simulink model "Parent_Mobile"  (R2023a)
settings: Solver=FixedStepDiscrete  StartTime=0.0  StopTime=inf  RelTol=1e-3
undefined symbols (not defined in the file): Alt, Child_Safety, Lat, Lon, ThingSpeak_X_Acc, X_Acc, X_Gyro, Y_Acc, Y_Gyro, Z_Acc, Z_Gyro
libraries: androidcommunicationlib x16, androiduilib x13, androidsensorlib x7, androidaudiovideolib x5
settings Model: Creator=dhart  LastModifiedBy=dhart
settings OptimizationCC: EnhancedBackFolding=on  PassReuseOutputArgsAs=Individual arguments  ZeroExternalMemoryAtStartup=off  ZeroInternalMemoryAtStartup=off  MaxStackSize=64  OptimizeBlockOrder=speed  DifferentSizesBufferReuse=on  OptimizationCustomize=off  EfficientTunableParamExpr=on
settings DebuggingCC: ParameterTunabilityLossMsg=error
settings HardwareCC: ProdBitPerPointer=32  ProdBitPerSizeT=32  ProdBitPerPtrDiffT=32  ProdLargestAtomicInteger=Long  ProdLargestAtomicFloat=Double  ProdWordSize=32  ProdHWDeviceType=ARM Compatible->ARM Cortex
settings SFSimCC: MATLABDynamicMemAlloc=off
settings RTWCC: Description=Embedded Coder  SystemTargetFile=ert.tlc  HardwareBoard=Android Device  TLCOptions="-aInlineSetEventsForThisBaseRateFcn=TLC_FALSE -aSuppressMultiTaskScheduler=TLC_FALSE  -aRateBasedStepFcn=0"  TemplateMakefile=ert_default_tmf  RTWVerbose=off  Toolchain=Android SDK/NDK Tools  BuildConfiguration=Faster Runs
settings CodeAppCC: ForceParamTrailComments=on  IgnoreCustomStorageClasses=off  OperatorAnnotations=on  SimulinkDataObjDesc=on  SFDataObjDesc=on  InsertBlockDesc=on

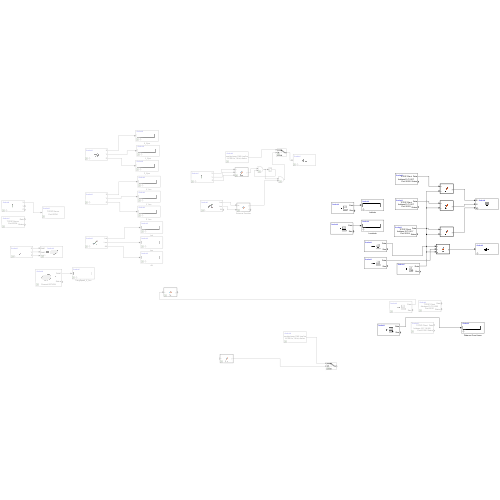
[thumbnail: Simulink's stored preview of the top-level diagram]
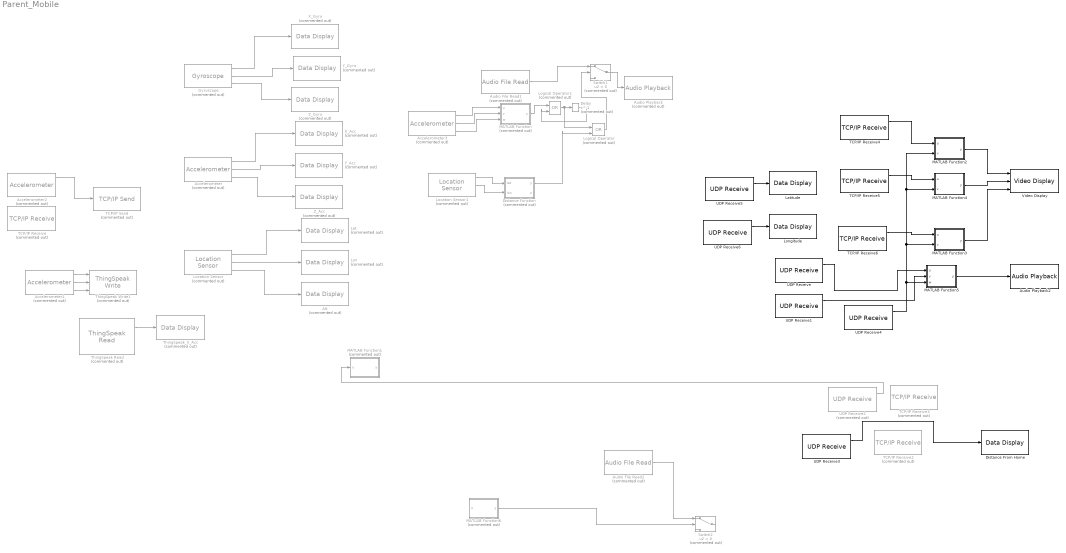
== system Parent_Mobile ==
  Accelerometer{,1..3} (4 alike) : androidsensorlib/Accelerometer  Commented=on  OutputVector=off  SampleTime=0.1  BlockPlatform=Android
  Alt : androiduilib/Data Display  Commented=on  DataDisplayId=Child_Safety/Alt  Format=Float  Precision=6  SimulateUsing=Code generation  blockPlatform=Android
  Audio File Read1 : androidaudiovideolib/Audio File Read  Commented=on  FileName=C:\Users\dhart\Downloads\mixkit-censorship-beep-1082 (mp3cut.net).wav  FrameSize=4410
  Audio File Read2 : androidaudiovideolib/Audio File Read  Commented=on  FileName=C:\Users\dhart\Downloads\mixkit-censorship-beep-1082 (mp3cut.net).wav  FrameSize=4410
  Audio Playback : androidaudiovideolib/Audio Playback  Commented=on  SampleFreq=44100  AudioSamplingFreq=44100  SampleTime=0.1  DeviceStr=0  QueueDuration=0  BlockPlatform=Android
  Audio Playback2 : androidaudiovideolib/Audio Playback  SampleFreq=44100  AudioSamplingFreq=44100  SampleTime=0.1  DeviceStr=0  QueueDuration=0  BlockPlatform=Android
  Delay : Delay  Commented=on  DelayLength=1  InitialCondition=0
  Distance From Home : androiduilib/Data Display  DataDisplayId=Parent_Mobile/Distance_From_Home  Format=Float  Precision=6  SimulateUsing=Code generation  blockPlatform=Android
  Distance Function : MATLAB Function  Commented=on  TreatAsAtomicUnit=on
  Gyroscope : androidsensorlib/Gyroscope  Commented=on  OutputVector=off  SampleTime=0.1  BlockPlatform=Android
  Lat : androiduilib/Data Display  Commented=on  DataDisplayId=Child_Safety/Lat  Format=Float  Precision=6  SimulateUsing=Code generation  blockPlatform=Android
  Latitude : androiduilib/Data Display  DataDisplayId=Parent_Mobile/Latitude  Format=Float  Precision=6  SimulateUsing=Code generation  blockPlatform=Android
  Location Sensor : androidsensorlib/Location Sensor  Commented=on  OutputVector=off  SampleTime=0.1  BlockPlatform=Android
  Location Sensor1 : androidsensorlib/Location Sensor  Commented=on  OutputVector=off  SampleTime=0.1  BlockPlatform=Android
  Logical Operator : Logic  Commented=on  Operator=OR  IconShape=distinctive  AllPortsSameDT=off  OutDataTypeStr=boolean
  Logical Operator1 : Logic  Commented=on  Operator=OR  IconShape=distinctive  AllPortsSameDT=off  OutDataTypeStr=boolean
  Lon : androiduilib/Data Display  Commented=on  DataDisplayId=Child_Safety/Lon  Format=Float  Precision=6  SimulateUsing=Code generation  blockPlatform=Android
  Longitude : androiduilib/Data Display  DataDisplayId=Parent_Mobile/Longitude  Format=Float  Precision=6  SimulateUsing=Code generation  blockPlatform=Android
  MATLAB Function : MATLAB Function  Commented=on  TreatAsAtomicUnit=on
  MATLAB Function1 : MATLAB Function  Commented=on  TreatAsAtomicUnit=on
  MATLAB Function2 : MATLAB Function  TreatAsAtomicUnit=on
  MATLAB Function3 : MATLAB Function  TreatAsAtomicUnit=on
  MATLAB Function4 : MATLAB Function  TreatAsAtomicUnit=on
  MATLAB Function5 : MATLAB Function  TreatAsAtomicUnit=on
  MATLAB Function6 : MATLAB Function  Commented=on  TreatAsAtomicUnit=on
  Switch1 : Switch  Commented=on  Criteria=u2 > Threshold  SaturateOnIntegerOverflow=off  InputSameDT=off
  Switch2 : Switch  Commented=on  Criteria=u2 > Threshold  SaturateOnIntegerOverflow=off  InputSameDT=off
  TCP/IP Receive : androidcommunicationlib/TCP//IP Receive  Commented=on  TCPReceiveId=Child_Safety/TCP//IP_Receive  Mode_=Server  LocalServerPort_=25784  RemoteAddr_=127.0.0.1  RemoteServerPort_=25000  DataType_=uint8  DataSize_=1  SampleTime_=0.1  ClientPortBindingSelection_=off  ClientPortToBind_=35000  BlockingMode_=off  BlockTimeout_=0.1
  TCP/IP Receive2 : androidcommunicationlib/TCP//IP Receive  Commented=on  TCPReceiveId=Parent_Mobile/TCP//IP_Receive2  Mode_=Client  LocalServerPort_=25000  RemoteAddr_=10.7.18.205  RemoteServerPort_=25150  DataType_=int16  DataSize_=1  SampleTime_=0.1  ClientPortBindingSelection_=off  ClientPortToBind_=35000  BlockingMode_=off  BlockTimeout_=0.1
  TCP/IP Receive3 : androidcommunicationlib/TCP//IP Receive  Commented=on  TCPReceiveId=Parent_Mobile/TCP//IP_Receive3  Mode_=Client  LocalServerPort_=25000  RemoteAddr_=10.7.18.205  RemoteServerPort_=25151  DataType_=int16  DataSize_=4410  SampleTime_=0.1  ClientPortBindingSelection_=off  ClientPortToBind_=35000  BlockingMode_=off  BlockTimeout_=0.1
  TCP/IP Receive4 : androidcommunicationlib/TCP//IP Receive  TCPReceiveId=Parent_Mobile/TCP//IP_Receive4  Mode_=Client  LocalServerPort_=25000  RemoteAddr_=10.7.2.217  RemoteServerPort_=39152  DataType_=uint8  DataSize_=76800  SampleTime_=2  ClientPortBindingSelection_=off  ClientPortToBind_=35000  BlockingMode_=off  BlockTimeout_=0.1
  TCP/IP Receive5 : androidcommunicationlib/TCP//IP Receive  TCPReceiveId=Parent_Mobile/TCP//IP_Receive5  Mode_=Client  LocalServerPort_=25000  RemoteAddr_=10.7.2.217  RemoteServerPort_=39153  DataType_=uint8  DataSize_=76800  SampleTime_=2  ClientPortBindingSelection_=off  ClientPortToBind_=35000  BlockingMode_=off  BlockTimeout_=0.1
  TCP/IP Receive6 : androidcommunicationlib/TCP//IP Receive  TCPReceiveId=Parent_Mobile/TCP//IP_Receive6  Mode_=Client  LocalServerPort_=25000  RemoteAddr_=10.7.2.217  RemoteServerPort_=39154  DataType_=uint8  DataSize_=76800  SampleTime_=2  ClientPortBindingSelection_=off  ClientPortToBind_=35000  BlockingMode_=off  BlockTimeout_=0.1
  TCP/IP Send : androidcommunicationlib/TCP//IP Send  Commented=on  TCPSendId=Child_Safety/TCP//IP_Send  Mode_=Server  LocalServerPort_=25784  RemoteAddr_=127.0.0.1  RemoteServerPort_=25498  ClientPortBindingSelection_=off  ClientPortToBind_=35000  BlockingMode_=off  BlockTimeout_=0.1
  ThingSpeak Read : androidcommunicationlib/ThingSpeak Read  Commented=on  ChannelID=2273034  ChannelAccess=Private  ReadAPIKey=WXUH9J7EYEMDF8NM  FieldNumber=1  SampleTime=0.1
  ThingSpeak Write1 : androidcommunicationlib/ThingSpeak Write  Commented=on  ChannelID=2273034  WriteAPIKey=W5LD3WN1B2LJ7SVE  NumberOfFields=3  UpdateInterval=15  LocationEnabled=off  LocationSource=Block dialog  BlockPlatform=Android
  ThingSpeak_X_Acc : androiduilib/Data Display  Commented=on  DataDisplayId=Child_Safety/ThingSpeak_X_Acc  Format=Float  Precision=6  SimulateUsing=Code generation  blockPlatform=Android
  UDP Receive : androidcommunicationlib/UDP Receive  localURL='0.0.0.0'  localPort=39155  remoteURL='0.0.0.0'  remotePort=-1  recvBufferSize=8192  signalDatatype=int16  dims=4410  isVarSize=off  showBlockingTime=off  blockingTime=0  sampletime=0.1  blockPlatform=Android
  UDP Receive1 : androidcommunicationlib/UDP Receive  localURL='0.0.0.0'  localPort=39156  remoteURL='0.0.0.0'  remotePort=-1  recvBufferSize=8192  signalDatatype=int16  dims=4410  isVarSize=off  showBlockingTime=off  blockingTime=0  sampletime=0.1  blockPlatform=Android
  UDP Receive2 : androidcommunicationlib/UDP Receive  Commented=on  localURL='0.0.0.0'  localPort=25151  remoteURL='0.0.0.0'  remotePort=-1  recvBufferSize=8192  signalDatatype=int16  dims=4410  isVarSize=off  showBlockingTime=off  blockingTime=0  sampletime=0.1  blockPlatform=Android
  UDP Receive3 : androidcommunicationlib/UDP Receive  localURL='0.0.0.0'  localPort=39150  remoteURL='0.0.0.0'  remotePort=-1  recvBufferSize=8192  signalDatatype=double  dims=1  isVarSize=off  showBlockingTime=off  blockingTime=0  sampletime=0.1  blockPlatform=Android
  UDP Receive4 : androidcommunicationlib/UDP Receive  localURL='0.0.0.0'  localPort=39157  remoteURL='0.0.0.0'  remotePort=-1  recvBufferSize=8192  signalDatatype=single  dims=1  isVarSize=off  showBlockingTime=off  blockingTime=0  sampletime=0.1  blockPlatform=Android
  UDP Receive5 : androidcommunicationlib/UDP Receive  localURL='0.0.0.0'  localPort=39158  remoteURL='0.0.0.0'  remotePort=-1  recvBufferSize=8192  signalDatatype=double  dims=1  isVarSize=off  showBlockingTime=off  blockingTime=0  sampletime=0.1  blockPlatform=Android
  UDP Receive6 : androidcommunicationlib/UDP Receive  localURL='0.0.0.0'  localPort=39159  remoteURL='0.0.0.0'  remotePort=-1  recvBufferSize=8192  signalDatatype=double  dims=1  isVarSize=off  showBlockingTime=off  blockingTime=0  sampletime=0.1  blockPlatform=Android
  Video Display : androidaudiovideolib/Video Display  BlockPlatform=Android
  X_Acc : androiduilib/Data Display  Commented=on  DataDisplayId=Child_Safety/X_Acc  Format=Float  Precision=6  SimulateUsing=Code generation  blockPlatform=Android
  X_Gyro : androiduilib/Data Display  Commented=on  DataDisplayId=Child_Safety/X_Gyro  Format=Float  Precision=6  SimulateUsing=Code generation  blockPlatform=Android
  Y_Acc : androiduilib/Data Display  Commented=on  DataDisplayId=Child_Safety/Y_Acc  Format=Float  Precision=6  SimulateUsing=Code generation  blockPlatform=Android
  Y_Gyro : androiduilib/Data Display  Commented=on  DataDisplayId=Child_Safety/Y_Gyro  Format=Float  Precision=6  SimulateUsing=Code generation  blockPlatform=Android
  Z_Acc : androiduilib/Data Display  Commented=on  DataDisplayId=Child_Safety/Z_Acc  Format=Float  Precision=6  SimulateUsing=Code generation  blockPlatform=Android
  Z_Gyro : androiduilib/Data Display  Commented=on  DataDisplayId=Child_Safety/Z_Gyro  Format=Float  Precision=6  SimulateUsing=Code generation  blockPlatform=Android
  wires:
  Accelerometer/1 -> X_Acc/1
  Accelerometer/2 -> Y_Acc/1
  Accelerometer/3 -> Z_Acc/1
  Location Sensor/2 -> Lon/1
  Location Sensor/3 -> Alt/1
  Gyroscope/1 -> X_Gyro/1
  Gyroscope/2 -> Y_Gyro/1
  Gyroscope/3 -> Z_Gyro/1
  Location Sensor/1 -> Lat/1
  Location Sensor1/1 -> Distance Function/1(lat)
  Location Sensor1/2 -> Distance Function/2(lon)
  Accelerometer1/1 -> ThingSpeak Write1/1
  Accelerometer1/2 -> ThingSpeak Write1/2
  Accelerometer1/3 -> ThingSpeak Write1/3
  Accelerometer2/1 -> TCP/IP Send/1
  ThingSpeak Read/1 -> ThingSpeak_X_Acc/1
  Accelerometer3/1 -> MATLAB Function/1(u)
  Accelerometer3/2 -> MATLAB Function/2(v)
  Accelerometer3/3 -> MATLAB Function/3(w)
  Audio File Read1/1 -> Switch1/1
  Switch1/1 -> Audio Playback/1
  Distance Function/1(y) -> Logical Operator/2
  Logical Operator/1 -> Switch1/2
  MATLAB Function/1(y) -> Logical Operator1/1
  Logical Operator1/1 -> Logical Operator/1, Delay/1
  Delay/1 -> Logical Operator1/2
  MATLAB Function2/1(y) -> Video Display/1
  MATLAB Function4/1(y) -> Video Display/2
  MATLAB Function3/1(y) -> Video Display/3
  MATLAB Function5/1(y) -> Audio Playback2/1
  UDP Receive/1 -> MATLAB Function5/1(u)
  UDP Receive1/1 -> MATLAB Function5/2(v)
  TCP/IP Receive4/1 -> MATLAB Function2/1(u)
  TCP/IP Receive5/1 -> MATLAB Function4/1(u)
  TCP/IP Receive6/1 -> MATLAB Function3/1(u)
  UDP Receive3/1 -> Distance From Home/1
  UDP Receive2/1 -> MATLAB Function1/1(u)
  UDP Receive5/1 -> Latitude/1
  UDP Receive6/1 -> Longitude/1
  UDP Receive4/1 -> MATLAB Function2/2(v), MATLAB Function4/2(v), MATLAB Function3/2(v), MATLAB Function5/3(w)
  MATLAB Function6/1(y) -> Switch2/2
  Audio File Read2/1 -> Switch2/1

== matlab function Parent_Mobile/MATLAB Function ==
  data: u input; y output; v input; w input
function y = fcn(u, v, w)
    if (u^2 + v^2 + w^2)^(1/2) > 15
        y = 1;
    else
        y = 0;
    end
end

== matlab function Parent_Mobile/Distance Function ==
  data: lat input; y output; lon input; z output
function [y,z]= fcn(lat, lon)
 % Haversine formula to calculate distance between two points on Earth
    R = 6371; % Earth's radius in kilometers
    radius = 0.1;
    lat1_rad = deg2rad(23.210406);
    lon1_rad = deg2rad(72.683669);
    lat2_rad = deg2rad(lat);
    lon2_rad = deg2rad(lon);
    dlat = lat2_rad - lat1_rad;
    dlon = lon2_rad - lon1_rad;
    a = sin(dlat/2)^2 + cos(lat1_rad) * cos(lat2_rad) * sin(dlon/2)^2;
    c = 2 * atan2(sqrt(a), sqrt(1-a));
    distance = R * c;
    z = distance;
    
    % Check if the distance is greater than the specified radius
    if distance > radius
        y = 1; % Point is outside the specified radius
    else
        y = 0; % Point is inside or on the specified radius
    end
end

== matlab function Parent_Mobile/MATLAB Function1 ==
  data: u input; y output
function y = fcn(u)
    y = [u,u];
end

== matlab function Parent_Mobile/MATLAB Function2 ==
  data: u input; y output; v input
function y = fcn(u,v)
    if v == 0
        y = uint8(zeros(320,240));
    else
    y = reshape(u, 320, 240);
   end
end

== matlab function Parent_Mobile/MATLAB Function3 ==
  data: u input; y output; v input
function y = fcn(u,v)
    if v == 0
        y = uint8(zeros(320,240));
    else
    y = reshape(u, 320, 240);
   end
end

== matlab function Parent_Mobile/MATLAB Function4 ==
  data: u input; y output; v input
function y = fcn(u,v)
    if v == 0
        y = uint8(zeros(320,240));
    else
    y = reshape(u, 320, 240);
   end
end

== matlab function Parent_Mobile/MATLAB Function5 ==
  data: u input; y output; v input; w input
function y = fcn(u, v,w)
    if w == 0
        y = int16(zeros(4410, 2));
    else
    y = [u, v];
   end
end

== matlab function Parent_Mobile/MATLAB Function6 ==
  data: u input; y output
function y = fcn(u)
    if u > 0.1
        y = 1;
    else 
        y = 0;
    end
end
